simulink model "UDPConnection"  (R2022b)
settings: configuration reference "WheelSimConfiguration" (kept outside this file)
libraries: slrealtimeutilitieslib x2, slrealtimeiplib x2
settings Model: Creator=ateay  LastModifiedBy=MOSA
settings ConfigSetRef: SourceName=WheelSimConfiguration  SourceLocation=Base Workspace

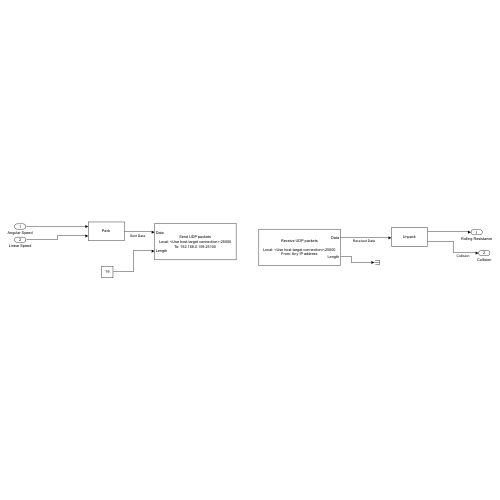
[thumbnail: Simulink's stored preview of the top-level diagram]
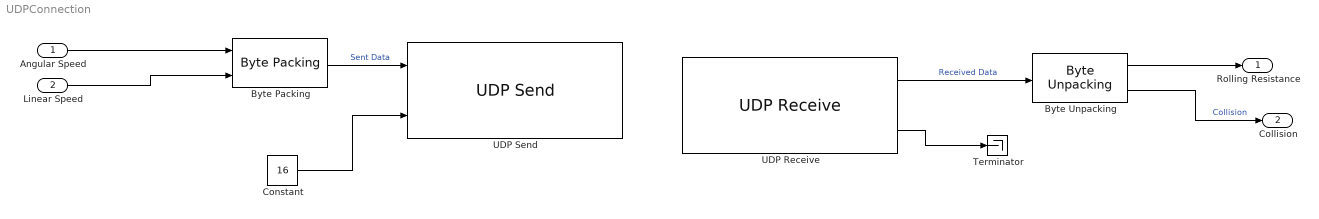
== system UDPConnection ==
  Angular Speed : Inport
  Linear Speed : Inport  Port=2
  Byte Packing : slrealtimeutilitieslib/Byte Packing  MaskPackedDataType=uint8  MaskUnpackedDataTypes={['double'],['double']}  MaskAlignment=1
  Byte Unpacking : slrealtimeutilitieslib/Byte Unpacking  MaskUnpackedDataTypes={['double'],'boolean'}  MaskUnpackedDataSizes={[1] [1]}  MaskAlignment=4
  Constant : Constant  Value=16
  Terminator : Terminator
  UDP Receive : slrealtimeiplib/UDP Receive  useHostTargetConn=on  ipAddress=192.168.0.200  localPort=25000  rcvWidth=12  rcvFmAny=on  fmAddress=192.168.0.2  sampleTime=simulator.TimeStep  enableMessage=off  maxPackets=1
  UDP Send : slrealtimeiplib/UDP Send  useHostTargetConn=on  toAddress=192.168.0.159  toPort=25100  sampleTime=simulator.TimeStep  enableMessage=off  ipAddress=192.168.0.200  localPort=25000
  Rolling Resistance : Outport
  Collision : Outport  Port=2
  wires:
  Byte Packing/1 -> UDP Send/1  "Sent Data"
  Angular Speed/1 -> Byte Packing/1
  Linear Speed/1 -> Byte Packing/2
  UDP Receive/1 -> Byte Unpacking/1  "Received Data"
  Constant/1 -> UDP Send/2
  UDP Receive/2 -> Terminator/1
  Byte Unpacking/1 -> Rolling Resistance/1
  Byte Unpacking/2 -> Collision/1  "Collision"
